simulink model "sim_ballAndPlate_complete"  (R2025a)
settings: Solver=FixedStepAuto  StartTime=0.0  StopTime=inf  FixedStep=0.001  RelTol=1e-3
values from neighbouring files (symbols this model uses):
  A_robust = [112.146929364 0.630225311398 -0.0528474836231 5.92800351843 -128.993499272 512.881237053 68.5135936991 -60.2481898853 -0.000560612606307 7.75681139646e-11 -8.40568260424e-14 3.63762304026e-12 ... (256 elements, 16x16)]    [optimalK.mat]    (also in setParams.m = K.A)
  B_robust = [8.71962327549e-06 2.66080283246e-08 -4.44588709662e-05 0.0249335751218 -0.124780550551 0.046876061655 -0.477448247916 0.125349385807 1.6391515998e-07 0.00789827917461 -0.0756062765532 0.0402835146702 ... (64 elements, 16x4)]    [optimalK.mat]    (also in setParams.m = K.B)
  Baw_robust = [-8.72218258115e-05 -0.00159732758501 -0.0086202709878 0.00368311983791 0.00078881186701 0.000275660317562 0.000337220649159 0.00123092844381 8.12455915287e-06 -8.60330482629e-11 -1.83473996813e-08 -3.69374837871e-08 ... (32 elements, 16x2)]    [optimalK.mat]    (also in setParams.m = C_robust' / (C_robust*C_robust' + aw_reg*eye(2)))
  C_robust = [-0.940288689094 2.07665990198e-10 -17.2198764127 3.87905252696e-09 -92.9302182263 -7.52432452741e-08 39.7056114333 0.000102247254523 8.50373022299 -0.00524029251965 2.97173645097 0.0202576810999 ... (32 elements, 2x16)]    [optimalK.mat]    (also in setParams.m = K.C)
  D_robust = [-7.30670123572e-08  2.49928002631e-05  -0.00101590554757  -103.887236737; 0.00101590546695  103.887238688  6.28490813402e-13  2.34910118024e-08]    [optimalK.mat]    (also in setParams.m = K.D)
  enable = 1    [setParams.m]
  g = 9.81    [setParams.m]
  G_B = G_A    [setParams.m]
  G_C = G_A    [setParams.m]
  I_max = 3    [setParams.m]
  inner_I_sat = 1    [setParams.m]
  K_lqr = dlqr(Ad, Bd, Q_lqr, R_lqr)    [setParams.m]
  Kaw_robust = 0.15    [optimalK.mat]    (also in setParams.m = 0.02)
  Km = 11    [setParams.m]
  m = m_a + 1/3 * m_p    (= 0.345333333333)    [setParams.m]
  Q_kf = diag([1, 100, 1, 100])    [setParams.m]
  r = 0.17    [PlateVisualizer.m]    (also in run_sim.m = squeeze(data.r.Data))
  R_kf = diag([0.1, 0.1])    [setParams.m]
  Ts_Inner = 0.001    [setParams.m]
  Ts_Outer = 1/50    (= 0.02)    [setParams.m]
  u_max_robust = [0.10471975512 0.10471975512]    [optimalK.mat]    (also in setParams.m = [ alpha_lim;  beta_lim])
  u_min_robust = [-0.10471975512 -0.10471975512]    [optimalK.mat]    (also in setParams.m = [-alpha_lim; -beta_lim])
  x0 = [0, 0, 0, 0]    [setParams.m]
  x_init = 0    [setParams.m]
  x_max = 0.03    [setParams.m]
undefined symbols (not defined in the file or in its folder): a, DiscIntNeverNeededParam, G_A
libraries: slpidlib x2, mpclib x1, simulink x1
settings Model: Creator=thoma  LastModifiedBy=thoma

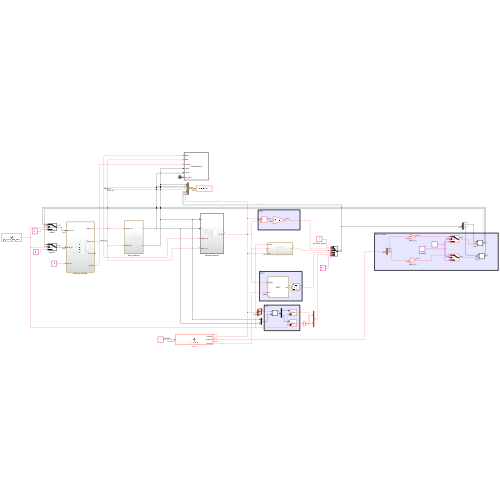
[thumbnail: Simulink's stored preview of the top-level diagram]
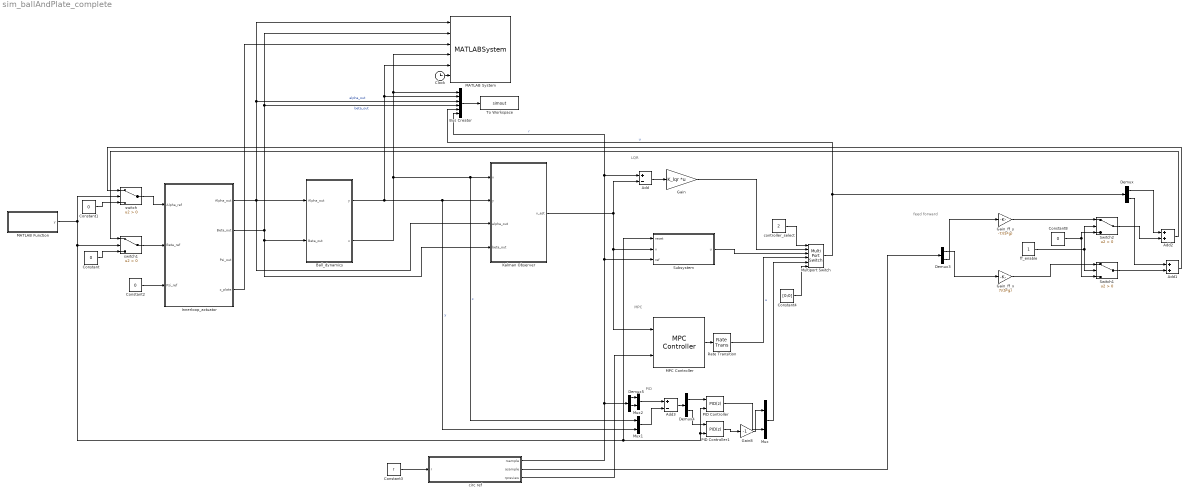
== system sim_ballAndPlate_complete ==
  note: LQR
  note: MPC
  note: feed forward
  note: PID
  Add : Sum  Inputs=+-
  Add1 : Sum
  Add2 : Sum
  Add3 : Sum  Inputs=+-
  Ball_dynamics : Subsystem
  Bus Creator : BusCreator  Inputs=6
  Clock : Clock
  Constant{,1..2,8} (4 alike) : Constant  Value=0
  Constant3 : Constant  Value=r
  Constant4 : Constant  Value=[0;0]
  Demux : Demux  Outputs=2
  Demux3 : Demux  Outputs=2
  Demux4 : Demux  Outputs=2
  Demux5 : Demux
  Gain : Gain  Gain=K_lqr  Multiplication=Matrix(K*u)
  Gain8 : Gain  Gain=-1
  Gain_ff_x : Gain  Gain=7/(5*g)
  "Gain_ff_y " : Gain  Gain=-7/(5*g)
  Innerloop_actuator : Subsystem
  Kalman Observer : Subsystem
  MATLAB Function : MATLAB Function  TreatAsAtomicUnit=on
  MATLAB System : MATLABSystem  System=PlateVisualizer  SimulateUsing=Code generation
      mask Type: PlateVisualizer
  MPC Controller : mpclib/MPC Controller  SCDEnableBlockLinearizationSpecification=on  mpcobj=mpcobj  is_multiple=0  enable_value=0  return_u0=off  updateMPCinCallerWorkspace=on  md_inport=off  mv_inport=off  uref_inport=off  return_cost=off  return_mvseq=off  return_qpstatus=off  return_xseq=off  return_state=off  return_ovseq=off  state_inport=on  umin_inport=off  umax_inport=off  ymin_inport=off  ymax_inport=off  cc_inport=off  ywt_inport=off  uwt_inport=off  duwt_inport=off  rhoeps_inport=off  pm_inport=off  MaximumP=10  HorizonChoice=FixedHorizon  n_ts=0.02  n_p=25  n_mv=2  n_md=0  n_ud=0  n_mo=4  n_uo=0  BlockDataType=double  SampleTimeInherited=off  switch_inport=off
  Multiport Switch : MultiPortSwitch  Inputs=5  SaturateOnIntegerOverflow=off  InputSameDT=off
  Mux : Mux  Inputs=2
  Mux1 : Mux  Inputs=2
  Mux2 : Mux  Inputs=2
  PID Controller : slpidlib/PID Controller  Controller=PID  Form=Parallel  TimeDomain=Discrete-time  UseExternalTs=off  SampleTime=-1  IntegratorMethod=Forward Euler  FilterMethod=Forward Euler  ControllerParametersSource=internal  P=0.6  I=0.08  UseKiTs=off  D=0.15  UseExternalDerivativeSource=off  N=25  UseFilter=on  TunerSelectOption=Transfer Function Based (PID Tuner App)  InitialConditionSource=internal  InitialConditionForIntegrator=0  InitialConditionForFilter=0  DifferentiatorICPrevScaledInput=0  ExternalReset=rising  TrackingMode=off  Kt=1  LimitOutput=off  SatLimitsSource=internal  UpperSaturationLimit=inf  LowerSaturationLimit=-inf  LinearizeAsGain=on  AntiWindupMode=none  Kb=1  LimitIntegrator=off  UpperIntegratorSaturationLimit=inf  LowerIntegratorSaturationLimit=-inf  POutMin=[]  POutMax=[]  IOutMin=[]  IOutMax=[]  DOutMin=[]  DOutMax=[]  NOutMin=[]  NOutMax=[]  SumOutMin=[]  SumOutMax=[]  SaturationOutMin=[]  SaturationOutMax=[]  PParamMin=[]  PParamMax=[]  IParamMin=[]  IParamMax=[]  DParamMin=[]  DParamMax=[]  NParamMin=[]  NParamMax=[]  KbParamMin=[]  KbParamMax=[]  KtParamMin=[]  KtParamMax=[]  KbOutMin=[]  KbOutMax=[]  KtOutMin=[]  KtOutMax=[]  IntegratorOutMin=[]  IntegratorOutMax=[]  FilterOutMin=[]  FilterOutMax=[]  SumI1OutMin=[]  SumI1OutMax=[]  SumI2OutMin=[]  SumI2OutMax=[]  SumI3OutMin=[]  SumI3OutMax=[]  SumI4OutMin=[]  SumI4OutMax=[]  SumDOutMin=[]  SumDOutMax=[]  DifferentiatorOutMin=[]  DifferentiatorOutMax=[]  FilterDiffOutCoefMin=[]  FilterDiffOutCoefMax=[]  ReciprocalOutMin=[]  ReciprocalOutMax=[]  SumDenOutMin=[]  SumDenOutMax=[]  SumNumOutMin=[]  SumNumOutMax=[]  DivideOutMin=[]  DivideOutMax=[]  UdiffTsProdOutMin=[]  UdiffTsProdOutMax=[]  NTsProdOutMin=[]  NTsProdOutMax=[]  UintegralTsProdOutMin=[]  UintegralTsProdOutMax=[]  UngainTsProdOutMin=[]  UngainTsProdOutMax=[]  ClampingZeroOutDataTypeStr=Inherit: Inherit via back propagation  ClampingZeroOutMin=[]  ClampingZeroOutMax=[]  FilterDenConstantOutDataTypeStr=Inherit: Inherit via back propagation  FilterDenConstantOutMin=[]  FilterDenConstantOutMax=[]  PCopyOutDataTypeStr=Inherit: Inherit via back propagation  PCopyOutMin=[]  PCopyOutMax=[]  NCopyOutDataTypeStr=Inherit: Inherit via back propagation  NCopyOutMin=[]  NCopyOutMax=[]  IntegratorContinuousStateAttributes=''  IntegratorStateMustResolveToSignalObject=off  IntegratorRTWStateStorageClass=Auto  FilterContinuousStateAttributes=''  FilterStateMustResolveToSignalObject=off  FilterRTWStateStorageClass=Auto  ParallelPVariant=InternalParameters  IdealPVariant=Disabled  IVariant=InternalParameters  DVariant=InternalParameters  IntegratorVariant=Discrete  SatVariant=Disabled  AWVariant=Passthrough  PCopyVariant=Disabled  TRVariant=Disabled  FdbkBlocksVariant=Forward  IdealPFdbkVariant=Disabled  SatFdbkVariant=Disabled  DerivativeFilterVariant=ForwardEulerFilter  NVariant=InternalParameters  NCopyVariant=Disabled  FilterICVariant=InternalICsFilter  IntegratorICVariant=InternalICs  ExternalResetVariant=ExternalReset  TRSumVariant=Passthrough  SumFdbkVariant=Disabled  SumVariant=Sum_PID  TsampFilterVariant=InternalTs  TsampNgainVariant=Passthrough  TsampIntegralVariant=Disabled_SignalSpec  ExternalSaturationOutDataTypeStr=Inherit: Same as second input  DerivativeSourceVariant=ErrorSignal  PreIntVariant=InternalPreInt
  PID Controller1 : slpidlib/PID Controller  Controller=PID  Form=Parallel  TimeDomain=Discrete-time  UseExternalTs=off  SampleTime=-1  IntegratorMethod=Forward Euler  FilterMethod=Forward Euler  ControllerParametersSource=internal  P=0.6  I=0.08  UseKiTs=off  D=0.15  UseExternalDerivativeSource=off  N=25  UseFilter=on  TunerSelectOption=Transfer Function Based (PID Tuner App)  InitialConditionSource=internal  InitialConditionForIntegrator=0  InitialConditionForFilter=0  DifferentiatorICPrevScaledInput=0  ExternalReset=rising  TrackingMode=off  Kt=1  LimitOutput=off  SatLimitsSource=internal  UpperSaturationLimit=inf  LowerSaturationLimit=-inf  LinearizeAsGain=on  AntiWindupMode=none  Kb=1  LimitIntegrator=off  UpperIntegratorSaturationLimit=inf  LowerIntegratorSaturationLimit=-inf  POutMin=[]  POutMax=[]  IOutMin=[]  IOutMax=[]  DOutMin=[]  DOutMax=[]  NOutMin=[]  NOutMax=[]  SumOutMin=[]  SumOutMax=[]  SaturationOutMin=[]  SaturationOutMax=[]  PParamMin=[]  PParamMax=[]  IParamMin=[]  IParamMax=[]  DParamMin=[]  DParamMax=[]  NParamMin=[]  NParamMax=[]  KbParamMin=[]  KbParamMax=[]  KtParamMin=[]  KtParamMax=[]  KbOutMin=[]  KbOutMax=[]  KtOutMin=[]  KtOutMax=[]  IntegratorOutMin=[]  IntegratorOutMax=[]  FilterOutMin=[]  FilterOutMax=[]  SumI1OutMin=[]  SumI1OutMax=[]  SumI2OutMin=[]  SumI2OutMax=[]  SumI3OutMin=[]  SumI3OutMax=[]  SumI4OutMin=[]  SumI4OutMax=[]  SumDOutMin=[]  SumDOutMax=[]  DifferentiatorOutMin=[]  DifferentiatorOutMax=[]  FilterDiffOutCoefMin=[]  FilterDiffOutCoefMax=[]  ReciprocalOutMin=[]  ReciprocalOutMax=[]  SumDenOutMin=[]  SumDenOutMax=[]  SumNumOutMin=[]  SumNumOutMax=[]  DivideOutMin=[]  DivideOutMax=[]  UdiffTsProdOutMin=[]  UdiffTsProdOutMax=[]  NTsProdOutMin=[]  NTsProdOutMax=[]  UintegralTsProdOutMin=[]  UintegralTsProdOutMax=[]  UngainTsProdOutMin=[]  UngainTsProdOutMax=[]  ClampingZeroOutDataTypeStr=Inherit: Inherit via back propagation  ClampingZeroOutMin=[]  ClampingZeroOutMax=[]  FilterDenConstantOutDataTypeStr=Inherit: Inherit via back propagation  FilterDenConstantOutMin=[]  FilterDenConstantOutMax=[]  PCopyOutDataTypeStr=Inherit: Inherit via back propagation  PCopyOutMin=[]  PCopyOutMax=[]  NCopyOutDataTypeStr=Inherit: Inherit via back propagation  NCopyOutMin=[]  NCopyOutMax=[]  IntegratorContinuousStateAttributes=''  IntegratorStateMustResolveToSignalObject=off  IntegratorRTWStateStorageClass=Auto  FilterContinuousStateAttributes=''  FilterStateMustResolveToSignalObject=off  FilterRTWStateStorageClass=Auto  ParallelPVariant=InternalParameters  IdealPVariant=Disabled  IVariant=InternalParameters  DVariant=InternalParameters  IntegratorVariant=Discrete  SatVariant=Disabled  AWVariant=Passthrough  PCopyVariant=Disabled  TRVariant=Disabled  FdbkBlocksVariant=Forward  IdealPFdbkVariant=Disabled  SatFdbkVariant=Disabled  DerivativeFilterVariant=ForwardEulerFilter  NVariant=InternalParameters  NCopyVariant=Disabled  FilterICVariant=InternalICsFilter  IntegratorICVariant=InternalICs  ExternalResetVariant=ExternalReset  TRSumVariant=Passthrough  SumFdbkVariant=Disabled  SumVariant=Sum_PID  TsampFilterVariant=InternalTs  TsampNgainVariant=Passthrough  TsampIntegralVariant=Disabled_SignalSpec  ExternalSaturationOutDataTypeStr=Inherit: Same as second input  DerivativeSourceVariant=ErrorSignal  PreIntVariant=InternalPreInt
  Rate Transition : RateTransition
  Subsystem : Subsystem
  Switch1 : Switch  Criteria=u2 > Threshold  SaturateOnIntegerOverflow=off  InputSameDT=off
  Switch2 : Switch  Criteria=u2 > Threshold  SaturateOnIntegerOverflow=off  InputSameDT=off
  To Workspace : ToWorkspace  VariableName=simout  SaveFormat=Timeseries  SampleTime=-1
  circ ref : MATLAB Function  TreatAsAtomicUnit=on
  controller_select : Constant  Value=2
  ff_enable : Constant
  switch : Switch  Criteria=u2 > Threshold  SaturateOnIntegerOverflow=off  InputSameDT=off
  switch1 : Switch  Criteria=u2 > Threshold  SaturateOnIntegerOverflow=off  InputSameDT=off
  wires:
  Constant2/1 -> Innerloop_actuator/3(Psi_ref)
  Innerloop_actuator/2(Beta_out) -> Kalman Observer/4(beta_out), Ball_dynamics/2(Beta_out), Bus Creator/4, MATLAB System/2  "beta_out"
  Innerloop_actuator/1(Alpha_out) -> MATLAB System/1, Bus Creator/3, Kalman Observer/3(alpha_out), Ball_dynamics/1(Alpha_out)  "alpha_out"
  Ball_dynamics/1(y) -> Bus Creator/2, MATLAB System/5, Mux1/2, Kalman Observer/2(y)  "y"
  Ball_dynamics/2(x) -> MATLAB System/4, Bus Creator/1, Mux1/1, Kalman Observer/1(x)  "x"
  MATLAB Function/1(y) -> switch1/2, Subsystem/1("reset "), PID Controller/2, PID Controller1/2, switch/2
  Add2/1 -> switch1/1
  switch1/1 -> Innerloop_actuator/2(Beta_ref)
  switch/1 -> Innerloop_actuator/1(Alpha_ref)
  Add1/1 -> switch/1
  Innerloop_actuator/4(z_plate) -> MATLAB System/3
  MPC Controller/1 -> Rate Transition/1
  Multiport Switch/1 -> Bus Creator/5, Demux/1  "u"
  Constant1/1 -> switch/3
  Constant/1 -> switch1/3
  Bus Creator/1 -> To Workspace/1
  Clock/1 -> MATLAB System/6
  circ ref/3(rpreview) -> MPC Controller/2
  Rate Transition/1 -> Multiport Switch/4  "u"
  controller_select/1 -> Multiport Switch/1
  Add/1 -> Gain/1
  Kalman Observer/1(x_est) -> Subsystem/2("x "), MPC Controller/1, Add/2
  Gain/1 -> Multiport Switch/2
  Constant3/1 -> circ ref/1(r)
  circ ref/1(rsample) -> Demux5/1, Subsystem/3("ref "), Add/1, Bus Creator/6  "r"
  "Gain_ff_y "/1 -> Switch2/1
  ff_enable/1 -> Switch1/2, Switch2/2
  Demux3/1 -> Gain_ff_x/1
  Switch1/1 -> Add1/2
  Gain_ff_x/1 -> Switch1/1
  Demux3/2 -> "Gain_ff_y "/1
  Constant8/1 -> Switch1/3, Switch2/3
  Switch2/1 -> Add2/2
  Demux/1 -> Add2/1
  Demux/2 -> Add1/1
  Constant4/1 -> Multiport Switch/6
  circ ref/2(asample) -> Demux3/1
  Mux2/1 -> Add3/1
  Demux4/2 -> PID Controller1/1
  PID Controller/1 -> Mux/2
  Demux4/1 -> PID Controller/1
  Add3/1 -> Demux4/1
  Gain8/1 -> Mux/1
  PID Controller1/1 -> Gain8/1
  Mux/1 -> Multiport Switch/5
  Demux5/3 -> Mux2/2
  Demux5/1 -> Mux2/1
  Mux1/1 -> Add3/2
  Subsystem/1(u) -> Multiport Switch/3

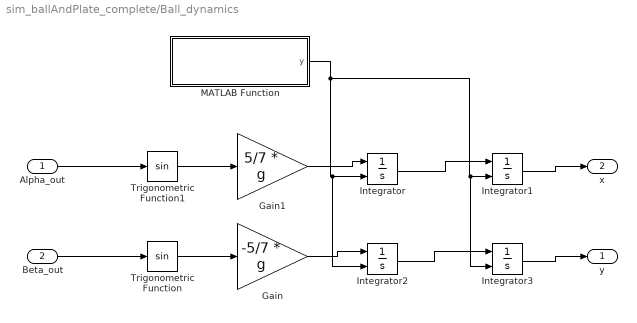
== system sim_ballAndPlate_complete/Ball_dynamics ==
  Alpha_out : Inport
  Beta_out : Inport  Port=2
  Gain : Gain  Gain=-5/7 * g
  Gain1 : Gain  Gain=5/7 * g
  Integrator : Integrator  ExternalReset=rising  InitialCondition=x0(2)
  Integrator1 : Integrator  ExternalReset=rising  InitialCondition=x0(1)
  Integrator2 : Integrator  ExternalReset=rising  InitialCondition=x0(4)
  Integrator3 : Integrator  ExternalReset=rising  InitialCondition=x0(2)
  MATLAB Function : MATLAB Function  TreatAsAtomicUnit=on
  Trigonometric Function : Trigonometry
  Trigonometric Function1 : Trigonometry
  y : Outport
  x : Outport  Port=2
  wires:
  Beta_out/1 -> Trigonometric Function/1
  Trigonometric Function/1 -> Gain/1
  Gain/1 -> Integrator2/1
  Trigonometric Function1/1 -> Gain1/1
  Alpha_out/1 -> Trigonometric Function1/1
  Gain1/1 -> Integrator/1
  Integrator/1 -> Integrator1/1
  Integrator1/1 -> x/1
  Integrator2/1 -> Integrator3/1
  Integrator3/1 -> y/1
  MATLAB Function/1(y) -> Integrator3/2, Integrator1/2, Integrator2/2, Integrator/2

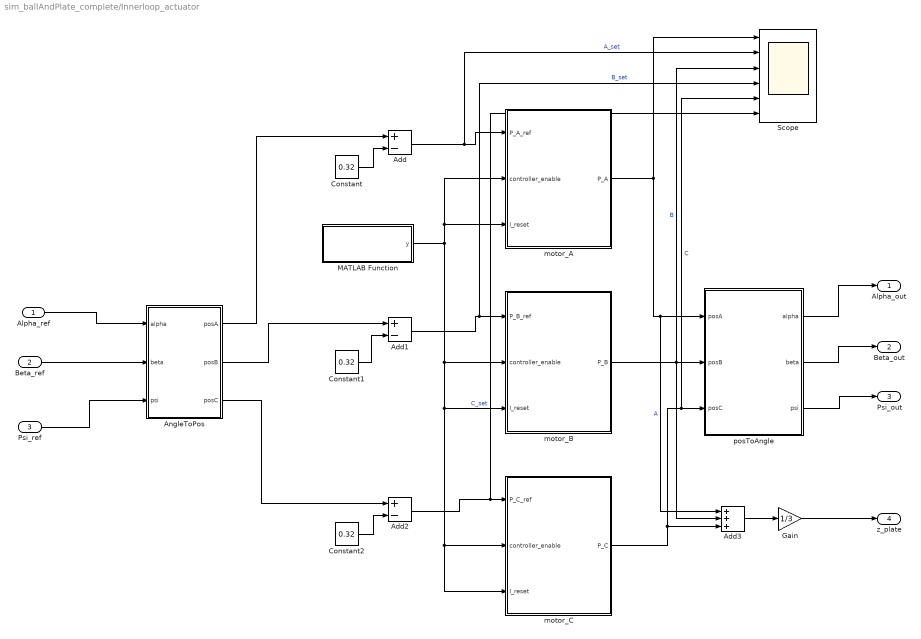
== system sim_ballAndPlate_complete/Innerloop_actuator ==
  Alpha_ref : Inport
  Beta_ref : Inport  Port=2
  Psi_ref : Inport  Port=3
  Add : Sum  Inputs=+-
  Add1 : Sum  Inputs=+-
  Add2 : Sum  Inputs=+-
  Add3 : Sum  Inputs=+++
  "AngleToPos " : MATLAB Function  TreatAsAtomicUnit=on
  Constant : Constant  Value=0.32
  Constant1 : Constant  Value=0.32
  Constant2 : Constant  Value=0.32
  Gain : Gain  Gain=1/3
  MATLAB Function : MATLAB Function  TreatAsAtomicUnit=on
  Scope : Scope  NumInputPorts=6
      settings: ActiveDisplayYMinimum=-0.0017528825710255869  ActiveDisplayYMaximum=0.0020437285369552553
  motor_A : Subsystem
  motor_B : Subsystem
  motor_C : Subsystem
  posToAngle : MATLAB Function  TreatAsAtomicUnit=on
  Alpha_out : Outport
  Beta_out : Outport  Port=2
  Psi_out : Outport  Port=3
  z_plate : Outport  Port=4
  wires:
  Alpha_ref/1 -> "AngleToPos "/1(alpha)
  Beta_ref/1 -> "AngleToPos "/2(beta)
  Psi_ref/1 -> "AngleToPos "/3(psi)
  Constant/1 -> Add/2
  Add/1 -> Scope/2, motor_A/1(P_A_ref)  "A_set"
  motor_A/1(P_A) -> Add3/1, posToAngle/1(posA), Scope/1  "A"
  "AngleToPos "/1(posA) -> Add/1
  posToAngle/1(alpha) -> Alpha_out/1
  "AngleToPos "/2(posB) -> Add1/1
  Add1/1 -> Scope/4, motor_B/1(P_B_ref)  "B_set"
  Constant1/1 -> Add1/2
  "AngleToPos "/3(posC) -> Add2/1
  Add2/1 -> Scope/6, motor_C/1(P_C_ref)  "C_set"
  Constant2/1 -> Add2/2
  motor_C/1(P_C) -> Add3/3, Scope/5, posToAngle/3(posC)  "C"
  motor_B/1(P_B) -> Scope/3, posToAngle/2(posB), Add3/2  "B"
  posToAngle/2(beta) -> Beta_out/1
  posToAngle/3(psi) -> Psi_out/1
  MATLAB Function/1(y) -> motor_B/3(I_reset), motor_C/3(I_reset), motor_C/2(controller_enable), motor_B/2(controller_enable), motor_A/3(I_reset), motor_A/2(controller_enable)
  Add3/1 -> Gain/1
  Gain/1 -> z_plate/1

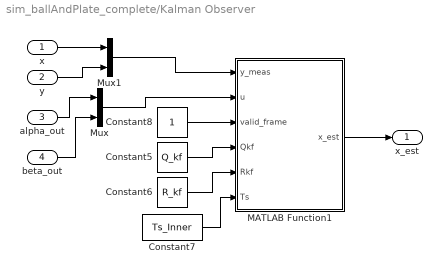
== system sim_ballAndPlate_complete/Kalman Observer ==
  x : Inport
  y : Inport  Port=2
  alpha_out : Inport  Port=3
  beta_out : Inport  Port=4
  Constant5 : Constant  Value=Q_kf
  Constant6 : Constant  Value=R_kf
  Constant7 : Constant  Value=Ts_Inner
  Constant8 : Constant
  MATLAB Function1 : MATLAB Function  TreatAsAtomicUnit=on
  Mux : Mux  Inputs=2
  Mux1 : Mux  Inputs=2
  x_est : Outport
  wires:
  Mux1/1 -> MATLAB Function1/1(y_meas)
  Constant7/1 -> MATLAB Function1/6(Ts)
  Constant5/1 -> MATLAB Function1/4(Qkf)
  x/1 -> Mux1/1
  Mux/1 -> MATLAB Function1/2(u)
  beta_out/1 -> Mux/2
  Constant8/1 -> MATLAB Function1/3(valid_frame)
  Constant6/1 -> MATLAB Function1/5(Rkf)
  MATLAB Function1/1(x_est) -> x_est/1
  y/1 -> Mux1/2
  alpha_out/1 -> Mux/1

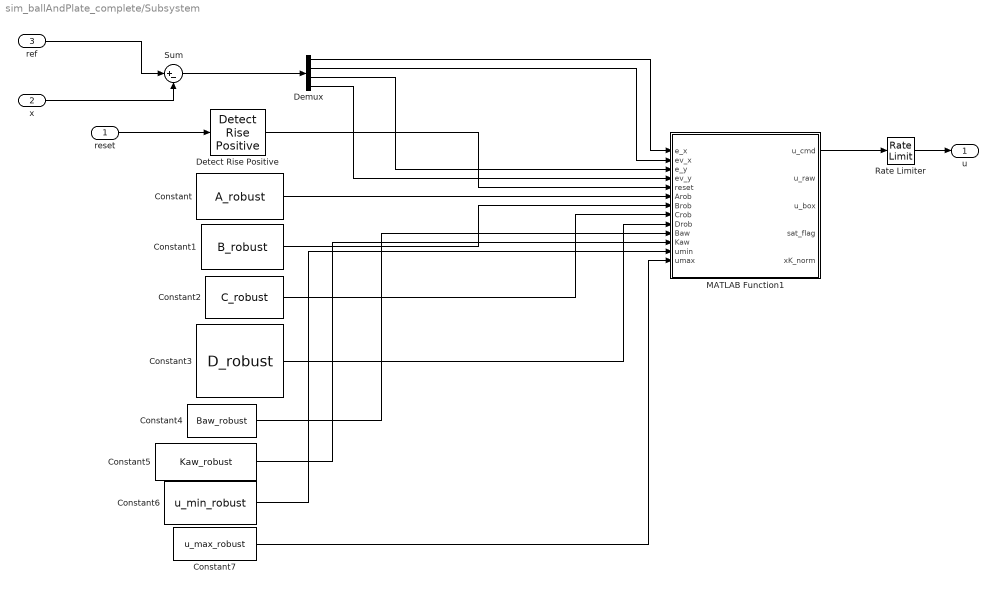
== system sim_ballAndPlate_complete/Subsystem ==
  "reset " : Inport
  "x " : Inport  Port=2
  "ref " : Inport  Port=3
  Constant : Constant  Value=A_robust  SampleTime=Ts_Outer
  Constant1 : Constant  Value=B_robust  SampleTime=Ts_Outer
  Constant2 : Constant  Value=C_robust  SampleTime=Ts_Outer
  Constant3 : Constant  Value=D_robust  SampleTime=Ts_Outer
  Constant4 : Constant  Value=Baw_robust  SampleTime=Ts_Outer
  Constant5 : Constant  Value=Kaw_robust  SampleTime=Ts_Outer
  Constant6 : Constant  Value=u_min_robust  SampleTime=Ts_Outer
  Constant7 : Constant  Value=u_max_robust  SampleTime=Ts_Outer
  Demux : Demux
  Detect Rise Positive : simulink/Logic and Bit Operations/Detect Rise Positive  vinit=0  OutDataTypeStr=boolean
  MATLAB Function1 : MATLAB Function  TreatAsAtomicUnit=on
  Rate Limiter : RateLimiter  RisingSlewLimit=deg2rad(12)  FallingSlewLimit=-deg2rad(12)  SampleTimeMode=inherited
  Sum : Sum  Inputs=|+-
  u : Outport
  wires:
  Constant/1 -> MATLAB Function1/6(Arob)
  Constant1/1 -> MATLAB Function1/7(Brob)
  Constant2/1 -> MATLAB Function1/8(Crob)
  Constant3/1 -> MATLAB Function1/9(Drob)
  Constant4/1 -> MATLAB Function1/10(Baw)
  Constant5/1 -> MATLAB Function1/11(Kaw)
  Constant6/1 -> MATLAB Function1/12(umin)
  Constant7/1 -> MATLAB Function1/13(umax)
  Detect Rise Positive/1 -> MATLAB Function1/5(reset)
  "reset "/1 -> Detect Rise Positive/1
  Demux/1 -> MATLAB Function1/1(e_x)
  Demux/2 -> MATLAB Function1/2(ev_x)
  Demux/3 -> MATLAB Function1/3(e_y)
  Demux/4 -> MATLAB Function1/4(ev_y)
  "ref "/1 -> Sum/1
  "x "/1 -> Sum/2
  Sum/1 -> Demux/1
  MATLAB Function1/1(u_cmd) -> Rate Limiter/1
  Rate Limiter/1 -> u/1

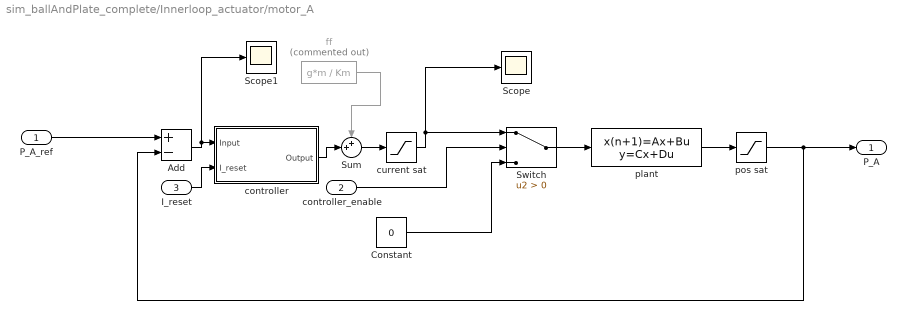
== system sim_ballAndPlate_complete/Innerloop_actuator/motor_A ==
  P_A_ref : Inport
  controller_enable : Inport  Port=2
  I_reset : Inport  Port=3
  Add : Sum  Inputs=+-
  Constant : Constant  Value=0
  Scope : Scope
      settings: ActiveDisplayYMinimum=-0.2151003532733422  ActiveDisplayYMaximum=0.78783772218945147  DataLoggingVariableName=ScopeData3
  Scope1 : Scope
      settings: ActiveDisplayYMinimum=-0.013802200769437761  ActiveDisplayYMaximum=0.022158674956348122  DataLoggingVariableName=ScopeData5
  Sum : Sum  Inputs=++|
  Switch : Switch  Criteria=u2 > Threshold  SaturateOnIntegerOverflow=off  InputSameDT=off
  controller : Subsystem
  current sat : Saturate  UpperLimit=I_max  LowerLimit=-I_max
  ff : Constant  Commented=on  Value=g*m / Km
  plant : DiscreteStateSpace  A=G_A.A  B=G_A.B  C=G_A.C  D=G_A.D  SampleTime=-1
  pos sat : Saturate  UpperLimit=x_max  LowerLimit=-x_max
  P_A : Outport
  wires:
  P_A_ref/1 -> Add/1
  controller/1(Output) -> Sum/2
  plant/1 -> pos sat/1
  pos sat/1 -> Add/2, P_A/1
  controller_enable/1 -> Switch/2
  current sat/1 -> Switch/1, Scope/1
  Switch/1 -> plant/1
  Constant/1 -> Switch/3
  Add/1 -> Scope1/1, controller/1(Input)
  I_reset/1 -> controller/2(I_reset)
  ff/1 -> Sum/1
  Sum/1 -> current sat/1

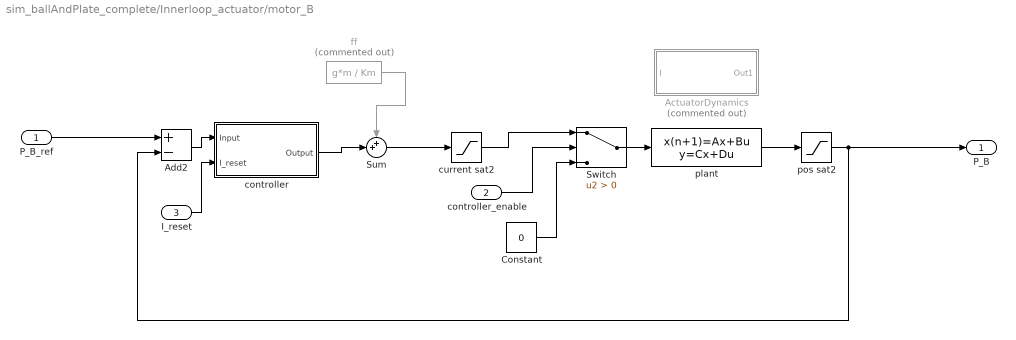
== system sim_ballAndPlate_complete/Innerloop_actuator/motor_B ==
  P_B_ref : Inport
  controller_enable : Inport  Port=2
  I_reset : Inport  Port=3
  ActuatorDynamics : Subsystem  Commented=on
  Add2 : Sum  Inputs=+-
  Constant : Constant  Value=0
  Sum : Sum  Inputs=++|
  Switch : Switch  Criteria=u2 > Threshold  SaturateOnIntegerOverflow=off  InputSameDT=off
  controller : Subsystem
  current sat2 : Saturate  UpperLimit=I_max  LowerLimit=-I_max
  ff : Constant  Commented=on  Value=g*m / Km
  plant : DiscreteStateSpace  A=G_B.A  B=G_B.B  C=G_B.C  D=G_B.D  SampleTime=-1
  pos sat2 : Saturate  UpperLimit=x_max  LowerLimit=-x_max
  P_B : Outport
  wires:
  controller_enable/1 -> Switch/2
  P_B_ref/1 -> Add2/1
  pos sat2/1 -> Add2/2, P_B/1
  Add2/1 -> controller/1(Input)
  controller/1(Output) -> Sum/2
  current sat2/1 -> Switch/1
  Constant/1 -> Switch/3
  ff/1 -> Sum/1
  Sum/1 -> current sat2/1
  Switch/1 -> plant/1
  plant/1 -> pos sat2/1
  I_reset/1 -> controller/2(I_reset)

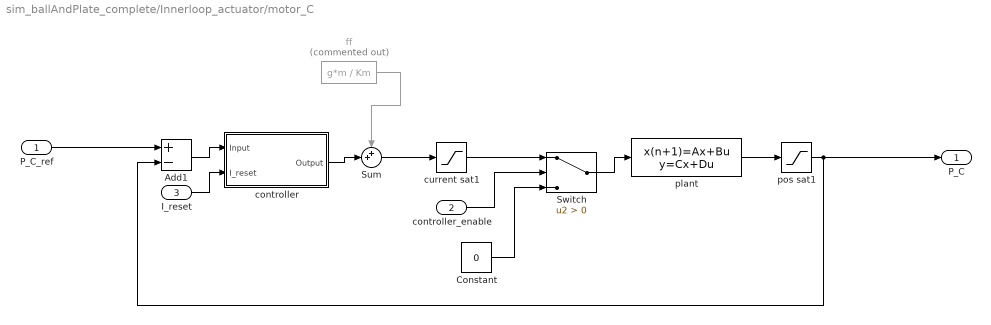
== system sim_ballAndPlate_complete/Innerloop_actuator/motor_C ==
  P_C_ref : Inport
  controller_enable : Inport  Port=2
  I_reset : Inport  Port=3
  Add1 : Sum  Inputs=+-
  Constant : Constant  Value=0
  Sum : Sum  Inputs=++|
  Switch : Switch  Criteria=u2 > Threshold  SaturateOnIntegerOverflow=off  InputSameDT=off
  controller : Subsystem
  current sat1 : Saturate  UpperLimit=I_max  LowerLimit=-I_max
  ff : Constant  Commented=on  Value=g*m / Km
  plant : DiscreteStateSpace  A=G_C.A  B=G_C.B  C=G_C.C  D=G_C.D  SampleTime=-1
  pos sat1 : Saturate  UpperLimit=x_max  LowerLimit=-x_max
  P_C : Outport
  wires:
  controller_enable/1 -> Switch/2
  Switch/1 -> plant/1
  plant/1 -> pos sat1/1
  P_C_ref/1 -> Add1/1
  pos sat1/1 -> Add1/2, P_C/1
  Add1/1 -> controller/1(Input)
  controller/1(Output) -> Sum/2
  current sat1/1 -> Switch/1
  Constant/1 -> Switch/3
  ff/1 -> Sum/1
  Sum/1 -> current sat1/1
  I_reset/1 -> controller/2(I_reset)

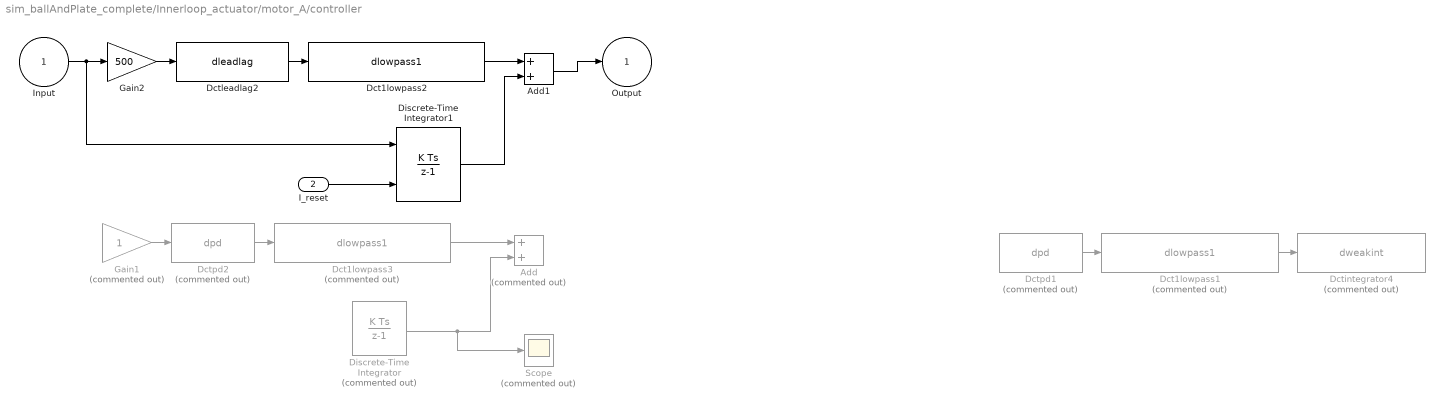
== system sim_ballAndPlate_complete/Innerloop_actuator/motor_A/controller ==
  Input : Inport
  I_reset : Inport  Port=2
  Add : Sum  Commented=on
  Add1 : Sum
  Dct1lowpass1 : S-Function  Commented=on  FunctionName=dlowpass1  Parameters=f_den, 0.001  SFunctionDeploymentMode=off  EnableBusSupport=off  mask(dctools){f_den=200}
      mask prompts: f_den "Pole [Hz]"
      mask help: This block implements a discrete time 1st order lowpass filter.
      mask Display: disp('DCT 1st order lowpass')
  Dct1lowpass2 : S-Function  FunctionName=dlowpass1  Parameters=f_den, 0.001  SFunctionDeploymentMode=off  EnableBusSupport=off  mask(dctools){f_den=50}
      mask prompts: f_den "Pole [Hz]"
      mask help: This block implements a discrete time 1st order lowpass filter.
      mask Display: disp('DCT 1st order lowpass')
  Dct1lowpass3 : S-Function  Commented=on  FunctionName=dlowpass1  Parameters=f_den, 0.001  SFunctionDeploymentMode=off  EnableBusSupport=off  mask(dctools){f_den=200}
      mask prompts: f_den "Pole [Hz]"
      mask help: This block implements a discrete time 1st order lowpass filter.
      mask Display: disp('DCT 1st order lowpass')
  Dctintegrator4 : S-Function  Commented=on  FunctionName=dweakint  Parameters=f_num, 0.001  SFunctionDeploymentMode=off  EnableBusSupport=off  mask(dctools){f_num=1}
      mask prompts: f_num "Zero [Hz]"
      mask help: This block implements a discrete time weak integrator filter.
      mask Display: disp('DCT integrator')
  Dctleadlag2 : S-Function  FunctionName=dleadlag  Parameters=f_num, f_den, 0.001  SFunctionDeploymentMode=off  EnableBusSupport=off  mask(dctools){f_num=7.5, f_den=30}
      mask prompts: f_num "Zero [Hz]"; f_den "Pole [Hz]"
      mask help: This block implements a discrete time leadlag filter.
      mask Display: disp('DCT leadlag')
  Dctpd1 : S-Function  Commented=on  FunctionName=dpd  Parameters=kp, kv, 0.001  SFunctionDeploymentMode=off  EnableBusSupport=off  mask(dctools){kp=0.01, kv=10}
      mask help: This block implements a discrete time pd filter.
      mask Display: disp('DCT pd')
  Dctpd2 : S-Function  Commented=on  FunctionName=dpd  Parameters=kp, kv, 0.001  SFunctionDeploymentMode=off  EnableBusSupport=off  mask(dctools){kp=0.01, kv=10}
      mask help: This block implements a discrete time pd filter.
      mask Display: disp('DCT pd')
  Discrete-Time Integrator : DiscreteIntegrator  Commented=on  gainval=1  ExternalReset=rising  SampleTime=-1  ICPrevOutput=DiscIntNeverNeededParam  ICPrevScaledInput=DiscIntNeverNeededParam
  Discrete-Time Integrator1 : DiscreteIntegrator  gainval=3531  ExternalReset=rising  SampleTime=-1  LimitOutput=on  UpperSaturationLimit=inner_I_sat  LowerSaturationLimit=-inner_I_sat  ICPrevOutput=DiscIntNeverNeededParam  ICPrevScaledInput=DiscIntNeverNeededParam
  Gain1 : Gain  Commented=on
  Gain2 : Gain  Gain=500  SaturateOnIntegerOverflow=on  OutDataTypeStr=Inherit: Same as input  ParamDataTypeStr=Inherit: Same as input
  Scope : Scope  Commented=on
      settings: ActiveDisplayYMinimum=-6.500387462094743E-17  ActiveDisplayYMaximum=0  DataLoggingVariableName=ScopeData8
  Output : Outport
  wires:
  Gain1/1 -> Dctpd2/1
  Dctpd2/1 -> Dct1lowpass3/1
  Dct1lowpass3/1 -> Add/1
  Discrete-Time Integrator/1 -> Scope/1, Add/2
  Dctpd1/1 -> Dct1lowpass1/1
  Dct1lowpass1/1 -> Dctintegrator4/1
  Input/1 -> Discrete-Time Integrator1/1, Gain2/1
  Discrete-Time Integrator1/1 -> Add1/2
  I_reset/1 -> Discrete-Time Integrator1/2
  Gain2/1 -> Dctleadlag2/1
  Dct1lowpass2/1 -> Add1/1
  Dctleadlag2/1 -> Dct1lowpass2/1
  Add1/1 -> Output/1

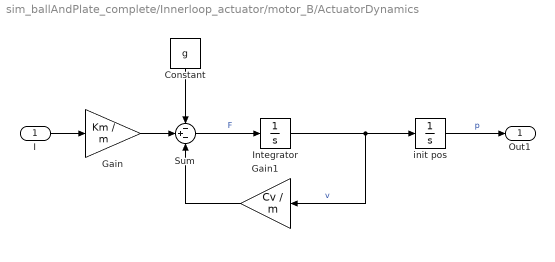
== system sim_ballAndPlate_complete/Innerloop_actuator/motor_B/ActuatorDynamics ==
  I : Inport
  Constant : Constant  Value=g
  Gain : Gain  Gain=Km / m
  Gain1 : Gain  Gain=Cv / m
  Integrator : Integrator
  Sum : Sum  Inputs=-+-
  init pos : Integrator  InitialCondition=x_init
  Out1 : Outport
  wires:
  I/1 -> Gain/1
  Gain/1 -> Sum/2
  init pos/1 -> Out1/1  "p"
  Sum/1 -> Integrator/1  "F"
  Integrator/1 -> Gain1/1, init pos/1  "v"
  Gain1/1 -> Sum/3
  Constant/1 -> Sum/1

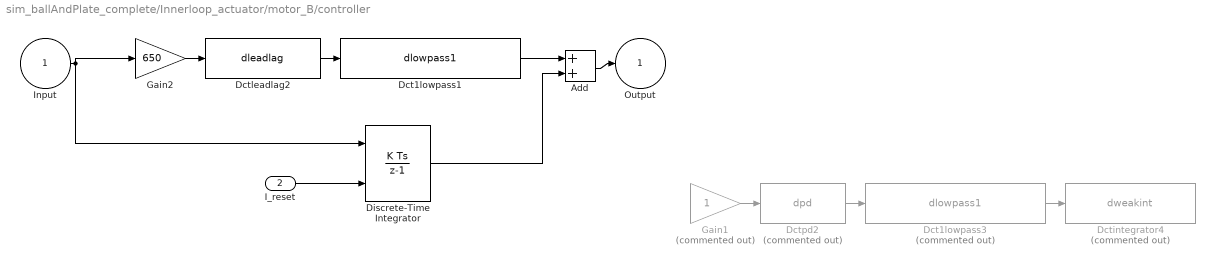
== system sim_ballAndPlate_complete/Innerloop_actuator/motor_B/controller ==
  Input : Inport
  I_reset : Inport  Port=2
  Add : Sum
  Dct1lowpass1 : S-Function  FunctionName=dlowpass1  Parameters=f_den, 0.001  SFunctionDeploymentMode=off  EnableBusSupport=off  mask(dctools){f_den=50}
      mask prompts: f_den "Pole [Hz]"
      mask help: This block implements a discrete time 1st order lowpass filter.
      mask Display: disp('DCT 1st order lowpass')
  Dct1lowpass3 : S-Function  Commented=on  FunctionName=dlowpass1  Parameters=f_den, 0.001  SFunctionDeploymentMode=off  EnableBusSupport=off  mask(dctools){f_den=200}
      mask prompts: f_den "Pole [Hz]"
      mask help: This block implements a discrete time 1st order lowpass filter.
      mask Display: disp('DCT 1st order lowpass')
  Dctintegrator4 : S-Function  Commented=on  FunctionName=dweakint  Parameters=f_num, 0.001  SFunctionDeploymentMode=off  EnableBusSupport=off  mask(dctools){f_num=1}
      mask prompts: f_num "Zero [Hz]"
      mask help: This block implements a discrete time weak integrator filter.
      mask Display: disp('DCT integrator')
  Dctleadlag2 : S-Function  FunctionName=dleadlag  Parameters=f_num, f_den, 0.001  SFunctionDeploymentMode=off  EnableBusSupport=off  mask(dctools){f_num=7.5, f_den=30}
      mask prompts: f_num "Zero [Hz]"; f_den "Pole [Hz]"
      mask help: This block implements a discrete time leadlag filter.
      mask Display: disp('DCT leadlag')
  Dctpd2 : S-Function  Commented=on  FunctionName=dpd  Parameters=kp, kv, 0.001  SFunctionDeploymentMode=off  EnableBusSupport=off  mask(dctools){kp=0.01, kv=10}
      mask help: This block implements a discrete time pd filter.
      mask Display: disp('DCT pd')
  Discrete-Time Integrator : DiscreteIntegrator  gainval=4102  ExternalReset=rising  SampleTime=-1  LimitOutput=on  UpperSaturationLimit=inner_I_sat  LowerSaturationLimit=-inner_I_sat  ICPrevOutput=DiscIntNeverNeededParam  ICPrevScaledInput=DiscIntNeverNeededParam
  Gain1 : Gain  Commented=on
  Gain2 : Gain  Gain=650  SaturateOnIntegerOverflow=on  OutDataTypeStr=Inherit: Same as input  ParamDataTypeStr=Inherit: Same as input
  Output : Outport
  wires:
  Gain1/1 -> Dctpd2/1
  Dctpd2/1 -> Dct1lowpass3/1
  Dct1lowpass3/1 -> Dctintegrator4/1
  Input/1 -> Gain2/1, Discrete-Time Integrator/1
  I_reset/1 -> Discrete-Time Integrator/2
  Discrete-Time Integrator/1 -> Add/2
  Dct1lowpass1/1 -> Add/1
  Gain2/1 -> Dctleadlag2/1
  Dctleadlag2/1 -> Dct1lowpass1/1
  Add/1 -> Output/1

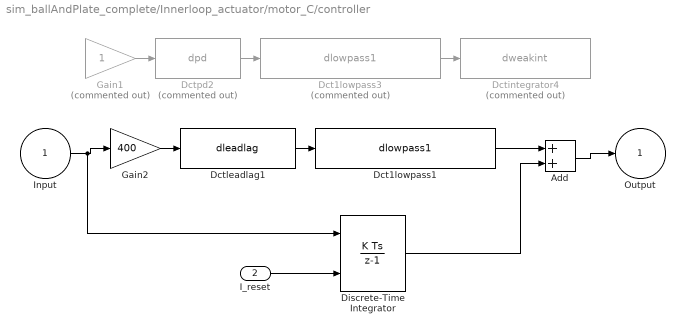
== system sim_ballAndPlate_complete/Innerloop_actuator/motor_C/controller ==
  Input : Inport
  I_reset : Inport  Port=2
  Add : Sum
  Dct1lowpass1 : S-Function  FunctionName=dlowpass1  Parameters=f_den, 0.001  SFunctionDeploymentMode=off  EnableBusSupport=off  mask(dctools){f_den=50}
      mask prompts: f_den "Pole [Hz]"
      mask help: This block implements a discrete time 1st order lowpass filter.
      mask Display: disp('DCT 1st order lowpass')
  Dct1lowpass3 : S-Function  Commented=on  FunctionName=dlowpass1  Parameters=f_den, 0.001  SFunctionDeploymentMode=off  EnableBusSupport=off  mask(dctools){f_den=200}
      mask prompts: f_den "Pole [Hz]"
      mask help: This block implements a discrete time 1st order lowpass filter.
      mask Display: disp('DCT 1st order lowpass')
  Dctintegrator4 : S-Function  Commented=on  FunctionName=dweakint  Parameters=f_num, 0.001  SFunctionDeploymentMode=off  EnableBusSupport=off  mask(dctools){f_num=1}
      mask prompts: f_num "Zero [Hz]"
      mask help: This block implements a discrete time weak integrator filter.
      mask Display: disp('DCT integrator')
  Dctleadlag1 : S-Function  FunctionName=dleadlag  Parameters=f_num, f_den, 0.001  SFunctionDeploymentMode=off  EnableBusSupport=off  mask(dctools){f_num=7.5, f_den=30}
      mask prompts: f_num "Zero [Hz]"; f_den "Pole [Hz]"
      mask help: This block implements a discrete time leadlag filter.
      mask Display: disp('DCT leadlag')
  Dctpd2 : S-Function  Commented=on  FunctionName=dpd  Parameters=kp, kv, 0.001  SFunctionDeploymentMode=off  EnableBusSupport=off  mask(dctools){kp=0.01, kv=10}
      mask help: This block implements a discrete time pd filter.
      mask Display: disp('DCT pd')
  Discrete-Time Integrator : DiscreteIntegrator  gainval=2500  ExternalReset=rising  SampleTime=-1  LimitOutput=on  UpperSaturationLimit=inner_I_sat  LowerSaturationLimit=-inner_I_sat  ICPrevOutput=DiscIntNeverNeededParam  ICPrevScaledInput=DiscIntNeverNeededParam
  Gain1 : Gain  Commented=on
  Gain2 : Gain  Gain=400  SaturateOnIntegerOverflow=on  OutDataTypeStr=Inherit: Same as input  ParamDataTypeStr=Inherit: Same as input
  Output : Outport
  wires:
  Gain1/1 -> Dctpd2/1
  Dctpd2/1 -> Dct1lowpass3/1
  Dct1lowpass3/1 -> Dctintegrator4/1
  Gain2/1 -> Dctleadlag1/1
  Input/1 -> Discrete-Time Integrator/1, Gain2/1
  I_reset/1 -> Discrete-Time Integrator/2
  Dct1lowpass1/1 -> Add/1
  Discrete-Time Integrator/1 -> Add/2
  Dctleadlag1/1 -> Dct1lowpass1/1
  Add/1 -> Output/1

== matlab function sim_ballAndPlate_complete/MATLAB Function ==
  data: y output
function y = get_outer_loop_state()
    % This block queries the base workspace live at every single sample step
    % We declare evalin as extrinsic so the code generator bypasses it
    coder.extrinsic('evalin');
    
    % Initialize a safe compiled default value
    state_val = 0.0; 
    
    % Safely read the value from the MATLAB base workspace
    state_val = evalin('base', 'outer_loop_enable');
    
    % Cast the value to a standard double output
    y = double(state_val);
end

== matlab function sim_ballAndPlate_complete/Innerloop_actuator/posToAngle ==
  data: posA input; alpha output; posB input; posC input; beta output; psi output
function [alpha, beta, psi] = posToAngle(posA, posB, posC)
    % Returns the angles resulting from the given position
    % note: the position should be relative from the actuators midpoint in the global frame

    % Physical Constants
    r = 0.17;                 % Radius to joints (m)
    h = 0.322;                % Resting height (m)
    theta = deg2rad(120);     % angle between bases (rad)

    % Reconstruction of the Plate Unit Vectors 
    % We find where the joints are in the world frame by using the inputs
    % If pos = 0.322, the joints are exactly T_height above the base.
    P1_global = [r; 0; h + posA];
    P2_global = [r*cos(theta); r*sin(theta); h + posB];
    P3_global = [r*cos(theta); -r*sin(theta); h + posC];

    % Find the center of the tilted plate
    % The average of the three joint positions gives the center of the motion plate
    center = (P1_global + P2_global + P3_global) / 3;

    % Vectors from the plate center to the joints
    % This isolates the tilt of the plate surface
    v1 = P1_global - center;
    v2 = P2_global - center;
    v3 = P3_global - center;

    % Compute Unit Vectors
    uX = v1 / norm(v1);             % Plate X-axis
    u_temp = cross(uX, v3);         % Temporary vector to find normal
    uZ = u_temp / norm(u_temp);     % Plate Z-axis (Normal)
    uY = cross(uZ, uX);             % Plate Y-axis

    % Extract Tait-Bryan Angles
    beta = asin(-uX(3));                            
    alpha = asin(uY(3) / sqrt(1 - uX(3)^2));       
    psi = asin(uX(2) / sqrt(1 - uX(3)^2));
end

== matlab function sim_ballAndPlate_complete/Innerloop_actuator/MATLAB Function ==
  data: y output
function y = get_inner_loop_state()
    % This block queries the base workspace live at every single sample step
    % We declare evalin as extrinsic so the code generator bypasses it
    coder.extrinsic('evalin');
    
    % Initialize a safe compiled default value
    state_val = 0.0; 
    
    % Safely read the value from the MATLAB base workspace
    state_val = evalin('base', 'inner_loop_enable');
    
    % Cast the value to a standard double output
    y = double(state_val);
end

== matlab function sim_ballAndPlate_complete/Ball_dynamics/MATLAB Function ==
  data: y output
function y = get_sim_reset_loop_state()
    % This block queries the base workspace live at every single sample step
    % We declare evalin as extrinsic so the code generator bypasses it
    coder.extrinsic('evalin');
    
    % Initialize a safe compiled default value
    state_val = 0.0; 
    
    % Safely read the value from the MATLAB base workspace
    state_val = evalin('base', 'sim_reset');
    
    % Cast the value to a standard double output
    y = double(state_val);
end

== matlab function sim_ballAndPlate_complete/Subsystem/MATLAB Function1 ==
  settings: updateMethod=DISCRETE
  data: e_x input; u_cmd output; ev_x input; e_y input; ev_y input; reset input; Arob input; Brob input; Crob input; Drob input; Baw input; Kaw input; umin input; umax input; u_raw output; u_box output; sat_flag output; xK_norm output
function [u_cmd, u_raw, u_box, sat_flag, xK_norm] = Hinf( ...
    e_x, ev_x, e_y, ev_y, ...
    reset, ...
    Arob, Brob, Crob, Drob, ...
    Baw, Kaw, ...
    umin, umax)
%#codegen
%
% Hinf controller with:
%   1) hard angle saturation
%   2) command rate limiting
%   3) anti-windup based on the ACTUAL command sent to the plant
%
% Inputs:
%   e_x, ev_x, e_y, ev_y = [r_x-x; -xdot; r_z-z; -zdot]
%   reset                = 1 when outer loop disabled
%
% Outputs:
%   u_cmd = final command to plant / AngleToPos
%   u_raw = unconstrained Hinf output
%   u_box = amplitude-saturated Hinf output before rate limit

persistent xK u_prev initialized

nK = size(Arob,1);

if isempty(initialized)
    xK = zeros(nK,1);
    u_prev = zeros(2,1);
    initialized = true;
end

u_raw = zeros(2,1);
u_box = zeros(2,1);
u_cmd = zeros(2,1);
sat_flag = false;
xK_norm = 0;

% Reset controller state while outer loop is off
if reset ~= 0
    xK = zeros(nK,1);
    u_prev = zeros(2,1);
    return;
end

%% Inputs to Hinf controller

yK = [e_x; ev_x; e_y; ev_y];

u_min = [umin(1); umin(2)];
u_max = [umax(1); umax(2)];

%% Raw Hinf command

u_raw = Crob*xK + Drob*yK;

%% Hard amplitude saturation

u_box = min(max(u_raw, u_min), u_max);

%% Rate limit the command sent to the plant

Ts_outer = 0.02;              % Hinf sample time [s]
maxRate  = deg2rad(20.0);    % [rad/s]

du_max = maxRate * Ts_outer;

du = u_box - u_prev;

du_limited = min(max(du, [-du_max; -du_max]), [du_max; du_max]);

u_cmd = u_prev + du_limited;

% Final safety saturation
u_cmd = min(max(u_cmd, u_min), u_max);

%% Anti-windup
% Use the actual plant command, not only the amplitude-saturated command.

du_aw = u_cmd - u_raw;

x_nom = Arob*xK + Brob*yK;
x_next = x_nom + Kaw*(Baw*du_aw);

% Numerical guard
if any(~isfinite(x_next)) || norm(x_next) > 1e8
    x_next = zeros(nK,1);
    u_cmd = zeros(2,1);
end

xK = x_next;
u_prev = u_cmd;

sat_flag = any(abs(u_cmd - u_raw) > 1e-10);
xK_norm = norm(xK);
end

== matlab function sim_ballAndPlate_complete/Innerloop_actuator/AngleToPos  ==
  data: alpha input; posA output; beta input; psi input; posB output; posC output
function [posA, posB, posC] = angleToPos(alpha, beta, psi)
    % Returns the actuator positions required to reach the desired angle
    % note: the position is absolute in the global frame

    % Physical Constants
    r = 0.17;           % Joint radius (m)
    h = [0; 0; 0.32];  % Resting height vector (m)
    
    % Joint positions on base and plate (equilateral triangle)
    % These match the definitions in your posToAngle function
    theta = [0, deg2rad(240), deg2rad(120)];
    B = [r*cos(theta); r*sin(theta); zeros(1,3)]; % Base joints (b_i)
    P = [r*cos(theta); r*sin(theta); zeros(1,3)]; % Plate joints (p_i)
    
    % Rotation Matrices (Yaw-Pitch-Roll order)
    Rz = [cos(psi) -sin(psi) 0; sin(psi) cos(psi) 0; 0 0 1];
    Ry = [cos(beta) 0 sin(beta); 0 1 0; -sin(beta) 0 cos(beta)];
    Rx = [1 0 0; 0 cos(alpha) -sin(alpha); 0 sin(alpha) cos(alpha)];
    R_BtoP = Rz * Ry * Rx; 
    
    % Compute absolute position for each motor
    % Motor 1
    l1_vec = h + (R_BtoP * P(:,1)) - B(:,1);
    posA = norm(l1_vec);
    
    % Motor 2
    l2_vec = h + (R_BtoP * P(:,2)) - B(:,2);
    posB = norm(l2_vec);
    
    % Motor 3
    l3_vec = h + (R_BtoP * P(:,3)) - B(:,3);
    posC = norm(l3_vec);
end

== matlab function sim_ballAndPlate_complete/Kalman Observer/MATLAB Function1 ==
  settings: updateMethod=DISCRETE
  data: y_meas input; u input; x_est output; valid_frame input; Qkf input; Rkf input; Ts input
function x_est = intermittent_kalman(y_meas, u, valid_frame, Qkf, Rkf, Ts)
    
    g = 9.81;
    Ad = [1, Ts, 0,0;
        0, 1, 0, 0;
        0, 0, 1, Ts;
        0, 0, 0, 1];

    Bd = [5/14 * g * Ts^2, 0;
        5/7 * g * Ts, 0;
        0, 5/14 * g * Ts^2;
        0, 5/7 * g * Ts];
    
    Cd = [1 0 0 0;
        0 0 1 0];


    % Persistent variables keep their state between sample steps
    persistent x_hat P
    
    % Initialization on the very first time step
    if isempty(x_hat)
        x_hat = zeros(4,1);
        P = eye(4) * 0.1;
    end
    
    % 1. Prediction Step (Always executes)
    x_pred = Ad * x_hat + Bd * u;
    P_pred = Ad * P * Ad' + Qkf;
    
    % 2. Correction Step (Conditional)
    if valid_frame > 0.5
        % Frame is valid: Run normal Kalman Correction
        S = Cd * P_pred * Cd' + Rkf;
        K = P_pred * Cd' / S; % Equivalent to P_pred * Cd' * inv(S)
        
        x_hat = x_pred + K * (y_meas - Cd * x_pred);
        lastxhatvalid = x_hat;
        P = (eye(4) - K * Cd) * P_pred;
    else
        % Frame was dropped: Skip correction, trust physics prediction
        x_hat = x_hat;
        P = P_pred;
    end
    
    % Output the current state estimate
    x_est = x_hat;
end

== matlab function sim_ballAndPlate_complete/circ ref ==
  data: r input double; rsample output double size=[4,1]; asample output double size=[2,1]; a parameter double; enable parameter double; rpreview output double size=[25, 4]
function [rsample, asample, rpreview] = ref_player(r, a, enable)
%#codegen
Npreview = 25; % number of samples preview for MPC

% Persistent variable to track the current sample index
persistent idx_ref;

% Initialize the index on the very first time step
if isempty(idx_ref)
    idx_ref = 1;
end

% Determine the total number of offline samples available
N_total = size(r, 2);

% Preallocate outputs for code generation stability
rsample = zeros(4, 1);
asample = zeros(2, 1);
% CHANGED: 25 rows (time steps), 4 columns (states)
rpreview = zeros(Npreview, 4); 

% --- Trajectory Generation Logic ---
if enable == 1
    % 1. Extract the current sample
    if idx_ref <= N_total
        rsample = r(:, idx_ref);
        asample = a(:, idx_ref);
    else
        % Hold the final sample if the trajectory ends but enable stays 1
        rsample = r(:, N_total);
        asample = a(:, N_total);
    end
    
    % 2. Extract the next Npreview samples for MPC
    for i = 1:Npreview
        preview_idx = idx_ref + i; 
        
        if preview_idx <= N_total
            % CHANGED: Assign transposed column [1x4] into row i
            rpreview(i, :) = r(:, preview_idx)'; 
        else
            % Zero-order hold: Pad with the last available reference state 
            rpreview(i, :) = r(:, N_total)';
        end
    end
    
    % 3. Advance the index for the next sample time (Ts)
    if idx_ref <= N_total
        idx_ref = idx_ref + 1;
    end
else
    % --- Reset / Idle State (enable == 0) ---
    % Keep index reset to the first sample
    idx_ref = 1; 
    
    % Output the initial conditions while waiting
    rsample = r(:, 1);
    asample = a(:, 1);
    
    % Provide a static look-ahead from the starting point
    for i = 1:Npreview
        if (1 + i) <= N_total
            % CHANGED: Transpose required here too
            rpreview(i, :) = r(:, 1 + i)';
        else
            rpreview(i, :) = r(:, N_total)';
        end
    end
end
